simulink model "regulator_PID_obiekt"  (R2014a)
settings: Solver=ode4  StartTime=0.0  StopTime=40  FixedStep=0.01  RelTol=1e-3
undefined symbols (not defined in the file or in its folder): martwa_strefa, T0
undefined symbols (not defined in the file): RTDAC4PCIBaseAddress
settings Model: CovSFcnEnable=on  Creator=Piotr  LastModifiedBy=Praca
settings OptimizationCC: SimCompilerOptimization=off
settings DebuggingCC: UnderspecifiedInitializationDetection=Classic  FrameProcessingCompatibilityMsg=error
settings RTWCC: RTWCompilerOptimization=off

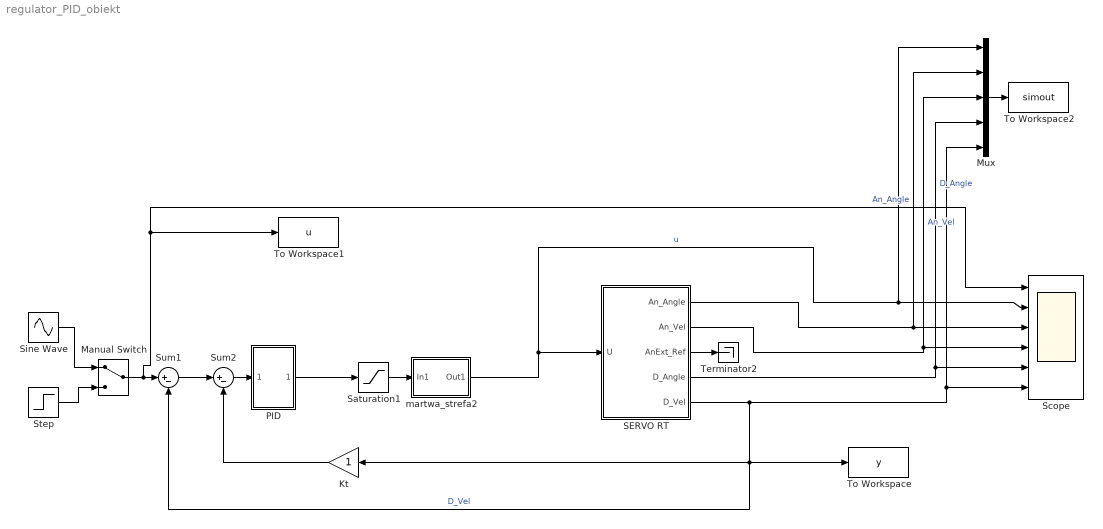
== system regulator_PID_obiekt ==
  Kt : Gain
  Manual Switch : ManualSwitch
  Mux : Mux  Inputs=5
  PID : Subsystem
  SERVO RT : Subsystem
  Saturation1 : Saturate  UpperLimit=1  LowerLimit=-1
  Scope : Scope  NumInputPorts=6
      settings: TimeRange=15  YMin=-0.493553~-4~0~0~0~-5  YMax=-0.446548~4~130~800~70~5  SaveName=obiekt  MaxDataPoints=40000  Decimation=2
  Sine Wave : Sin  SampleTime=0
  Step : Step  After=10  SampleTime=0
  Sum1 : Sum  Inputs=|+-
  Sum2 : Sum  Inputs=|+-
  Terminator2 : Terminator
  To Workspace : ToWorkspace  VariableName=y  SaveFormat=Structure With Time  SampleTime=-1
  To Workspace1 : ToWorkspace  VariableName=u  SaveFormat=Structure With Time  SampleTime=-1
  To Workspace2 : ToWorkspace  VariableName=simout  SaveFormat=Timeseries  SampleTime=-1
  martwa_strefa2 : Subsystem
  wires:
  Sine Wave/1 -> Manual Switch/1
  Step/1 -> Manual Switch/2
  PID/1(Out1) -> Saturation1/1
  Kt/1 -> Sum2/2
  Sum2/1 -> PID/1(In1)
  Sum1/1 -> Sum2/1
  Manual Switch/1 -> To Workspace1/1, Scope/1, Sum1/1
  Saturation1/1 -> martwa_strefa2/1(In1)
  SERVO RT/3(AnExt_Ref) -> Terminator2/1
  SERVO RT/1(An_Angle) -> Scope/3, Mux/2  "An_Angle"
  SERVO RT/2(An_Vel) -> Scope/4, Mux/3  "An_Vel"
  SERVO RT/4(D_Angle) -> Scope/5, Mux/4  "D_Angle"
  SERVO RT/5(D_Vel) -> To Workspace/1, Sum1/2, Kt/1, Scope/6, Mux/5  "D_Vel"
  martwa_strefa2/1(Out1) -> SERVO RT/1(U), Scope/2, Mux/1  "u"
  Mux/1 -> To Workspace2/1

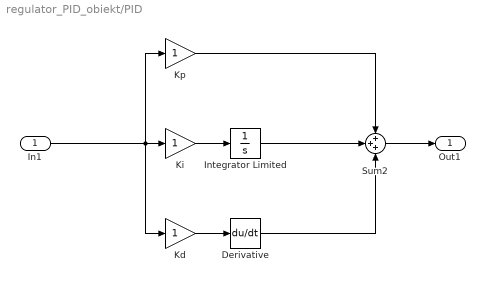
== system regulator_PID_obiekt/PID ==
  In1 : Inport
  Derivative : Derivative
  Integrator Limited : Integrator  LimitOutput=on  UpperSaturationLimit=1  LowerSaturationLimit=-1
  Kd : Gain
  Ki : Gain
  Kp : Gain
  Sum2 : Sum  Inputs=+++
  Out1 : Outport
  wires:
  Kp/1 -> Sum2/1
  Ki/1 -> Integrator Limited/1
  Sum2/1 -> Out1/1
  Kd/1 -> Derivative/1
  In1/1 -> Kp/1, Kd/1, Ki/1
  Derivative/1 -> Sum2/3
  Integrator Limited/1 -> Sum2/2

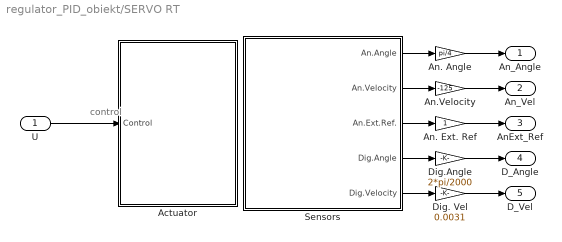
== system regulator_PID_obiekt/SERVO RT ==
  note: control
  U : Inport
  Actuator : Subsystem  mask(Servo Input){BaseAddr=RTDAC4PCIBaseAddress, T0=T0}
      mask prompts: BaseAddr "Base Address"; T0 "Sample Time"
      mask help: RTDAC/PCI Device Driver
      mask Display:
      | plot(0,0,55,85,[15,50,50,50,50,50,50,50,50,50,50,50,50,50,15,25,15],[100,100,90,80,75,70,60,50,40,30,25,20,10,0,0,50,100],[15,25],[50,50],[0,0],[20,80]);
      | text(30,47,'ES 151')
      | text(20,7,'RTDAC/PCI')
  An. Angle : Gain  Gain=pi/4  SaturateOnIntegerOverflow=on  OutDataTypeStr=Inherit: Same as input  ParamDataTypeStr=Inherit: Same as input
  An. Ext. Ref : Gain  SaturateOnIntegerOverflow=on  OutDataTypeStr=Inherit: Same as input  ParamDataTypeStr=Inherit: Same as input
  An.Velocity : Gain  Gain=-125  SaturateOnIntegerOverflow=on  OutDataTypeStr=Inherit: Same as input  ParamDataTypeStr=Inherit: Same as input
  Dig. Vel : Gain  Gain=0.0031  SaturateOnIntegerOverflow=on  OutDataTypeStr=Inherit: Same as input  ParamDataTypeStr=Inherit: Same as input
  Dig.Angle : Gain  Gain=2*pi/2000  SaturateOnIntegerOverflow=on  OutDataTypeStr=Inherit: Same as input  ParamDataTypeStr=Inherit: Same as input
  "Sensors                      " : Subsystem  mask(TRMS Output){BaseAddr=RTDAC4PCIBaseAddress, T0=T0}
      mask prompts: BaseAddr "Base address"; T0 "Sample Time"
      mask help: PCL-812 PG Device Driver
      mask Display:
      | plot(0,0,55,85,85-[55,80,80,80,80,80,80,80,80,80,80,80,80,80,55,50,55],[100,100,90,80,75,70,60,50,40,30,25,20,10,0,0,50,100],[55,55],[100,0],[54,55],[50,50]);
      | text(15,47,'ES 151')
      | text(10,7,'RTDAC/PCI')
  An_Angle : Outport
  An_Vel : Outport  Port=2
  AnExt_Ref : Outport  Port=3
  D_Angle : Outport  Port=4
  D_Vel : Outport  Port=5
  wires:
  An. Angle/1 -> An_Angle/1
  An. Ext. Ref/1 -> AnExt_Ref/1
  Dig. Vel/1 -> D_Vel/1
  An.Velocity/1 -> An_Vel/1
  U/1 -> Actuator/1(Control)
  Dig.Angle/1 -> D_Angle/1
  "Sensors                      "/5(Dig.Velocity) -> Dig. Vel/1
  "Sensors                      "/4(Dig.Angle) -> Dig.Angle/1
  "Sensors                      "/2(An.Velocity) -> An.Velocity/1
  "Sensors                      "/1(An.Angle) -> An. Angle/1
  "Sensors                      "/3(An.Ext.Ref.) -> An. Ext. Ref/1

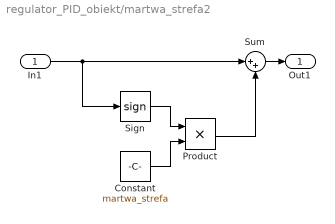
== system regulator_PID_obiekt/martwa_strefa2 ==
  In1 : Inport
  Constant : Constant  Value=martwa_strefa
  Product : Product
  Sign : Signum
  Sum : Sum  Inputs=|++
  Out1 : Outport
  wires:
  In1/1 -> Sum/1, Sign/1
  Product/1 -> Sum/2
  Sign/1 -> Product/1
  Constant/1 -> Product/2
  Sum/1 -> Out1/1

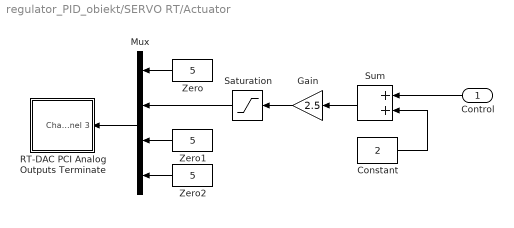
== system regulator_PID_obiekt/SERVO RT/Actuator ==
  Control : Inport
  Constant : Constant  Value=2
  Gain : Gain  Gain=2.5  OutDataTypeStr=Inherit: Same as input  ParamDataTypeStr=Inherit: Same as input
  Mux : Mux
  RT-DAC PCI Analog Outputs Terminate : Subsystem  mask(Analog Output Module){BaseAddress=RTDAC4PCIBaseAddress, VoltRange=-10V - +10V, SetOutputsFlag=on, SetOutputsValue=[0 5 0 0], T0=T0}
      mask prompts: BaseAddress "Base Address:"; VoltRange "Voltage Range"; SetOutputsFlag "Set Outputs At Termination"; SetOutputsValue "Termination Outputs [V]:"; T0 "Sample Time (sec):"
      mask help: RT-DAC PCI Device Driver
      mask Help: Set up each field for your specific hardware configuration.
      mask TypeOptions VoltRange: 0V - +10V | -10V - 0V | -10V - +10V
      mask Display: plot(0,0,100,100,[90,80,80,11,11],[90,90,20,20,80],[11,80],[80,80],[80,80],[20,14],[80,85,85,80],[45,45,66,66],[45,45,74,74],[20,13,13,20],[15,27,27,15,15],[75,75,26,26,75],[33,48,48,33,33],[75,75,55,55,75],[55,55,71,71,55],[55,75,75,55,55],[33,41,41,33,33],[50,50,27,27,50],[48,56,56,48,48],[50,50,27,27,50],[62,70,70,62,62],[50,50,27,27,50])
  Saturation : Saturate  UpperLimit=7.5  LowerLimit=2.5
  Sum : Sum  SaturateOnIntegerOverflow=on  InputSameDT=on  OutDataTypeStr=Inherit: Same as first input
  Zero : Constant  Value=5
  Zero1 : Constant  Value=5
  Zero2 : Constant  Value=5
  wires:
  Constant/1 -> Sum/2
  Sum/1 -> Gain/1
  Gain/1 -> Saturation/1
  Zero1/1 -> Mux/3
  Zero2/1 -> Mux/4
  Mux/1 -> RT-DAC PCI Analog Outputs Terminate/1(Channel 0 Channel 1 Channel 2 Channel 3)
  Saturation/1 -> Mux/2
  Zero/1 -> Mux/1
  Control/1 -> Sum/1

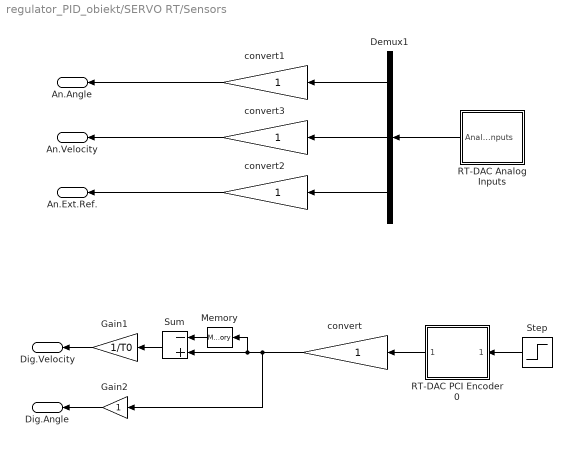
== system regulator_PID_obiekt/SERVO RT/Sensors                       ==
  Demux1 : Demux  Outputs=3
  Gain1 : Gain  Gain=1/T0  SaturateOnIntegerOverflow=on  OutDataTypeStr=Inherit: Same as input  ParamDataTypeStr=Inherit: Same as input
  Gain2 : Gain  SaturateOnIntegerOverflow=on  OutDataTypeStr=Inherit: Same as input  ParamDataTypeStr=Inherit: Same as input
  Memory : Memory
  RT-DAC Analog Inputs : Subsystem  mask(Analog Input Module){BaseAddress=RTDAC4PCIBaseAddress, Chan=[10 11 12], Gain=[1 1 1], T0=T0}
      mask prompts: BaseAddress "Base Address:"; Chan "Channel:"; T0 "Sample Time (sec):"
      mask help: RT-DAC PCI Device Driver
      mask Help: Set up each field for your specific hardware configuration.
      mask Display: plot(0,0,100,100,[90,80,80,11,11],[90,90,20,20,80],[11,80],[80,80],[80,80],[20,14],[80,85,85,80],[45,45,66,66],[45,45,74,74],[20,13,13,20],[15,27,27,15,15],[75,75,26,26,75],[33,48,48,33,33],[75,75,55,55,75],[55,55,71,71,55],[55,75,75,55,55],[33,41,41,33,33],[50,50,27,27,50],[48,56,56,48,48],[50,50,27,27,50],[62,70,70,62,62],[50,50,27,27,50])
  "RT-DAC PCI Encoder 0  " : Subsystem  mask(Incremental Encoders){BaseAddress=RTDAC4PCIBaseAddress, ChannelIdx=0, T0=T0}
      mask prompts: BaseAddress "Base Address:"; ChannelIdx "Channel:"; T0 "Sample Time (sec):"
      mask help: RT-DAC PCI Device Driver
      mask Help: Set up each field for your specific hardware configuration.
      mask TypeOptions ChannelIdx: 0 | 1 | 2 | 3
      mask Display: plot(0,0,100,100,[90,80,80,11,11],[90,90,20,20,80],[11,80],[80,80],[80,80],[20,14],[80,85,85,80],[45,45,66,66],[45,45,74,74],[20,13,13,20],[15,27,27,15,15],[75,75,26,26,75],[33,48,48,33,33],[75,75,55,55,75],[55,55,71,71,55],[55,75,75,55,55],[33,41,41,33,33],[50,50,27,27,50],[48,56,56,48,48],[50,50,27,27,50],[62,70,70,62,62],[50,50,27,27,50])
  Step : Step  Time=T0  Before=1  After=0  SampleTime=0
  Sum : Sum  Inputs=-+  SaturateOnIntegerOverflow=on  InputSameDT=on  OutDataTypeStr=Inherit: Same as first input
  convert : Gain  SaturateOnIntegerOverflow=on  OutDataTypeStr=Inherit: Same as input  ParamDataTypeStr=Inherit: Same as input
  convert1 : Gain  SaturateOnIntegerOverflow=on  OutDataTypeStr=Inherit: Same as input  ParamDataTypeStr=Inherit: Same as input
  convert2 : Gain  SaturateOnIntegerOverflow=on  OutDataTypeStr=Inherit: Same as input  ParamDataTypeStr=Inherit: Same as input
  convert3 : Gain  OutDataTypeStr=Inherit: Same as input  ParamDataTypeStr=Inherit: Same as input
  An.Angle : Outport  InitialOutput=0
  An.Velocity : Outport  Port=2  InitialOutput=0
  An.Ext.Ref. : Outport  Port=3  InitialOutput=0
  Dig.Angle : Outport  Port=4  InitialOutput=0
  Dig.Velocity : Outport  Port=5  InitialOutput=0
  wires:
  Step/1 -> "RT-DAC PCI Encoder 0  "/1(Reset)
  "RT-DAC PCI Encoder 0  "/1(Encoder Counter) -> convert/1
  convert3/1 -> An.Velocity/1
  Demux1/2 -> convert3/1
  convert2/1 -> An.Ext.Ref./1
  Demux1/3 -> convert2/1
  Gain2/1 -> Dig.Angle/1
  Sum/1 -> Gain1/1
  convert/1 -> Gain2/1, Sum/2, Memory/1
  Memory/1 -> Sum/1
  convert1/1 -> An.Angle/1
  Demux1/1 -> convert1/1
  RT-DAC Analog Inputs/1(Analog Inputs) -> Demux1/1
  Gain1/1 -> Dig.Velocity/1

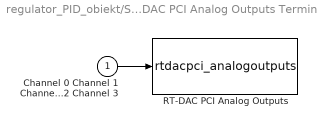
== system regulator_PID_obiekt/SERVO RT/Actuator/RT-DAC PCI Analog Outputs Terminate ==
  Channel 0 Channel 1 Channel 2 Channel 3 : Inport
  "RT-DAC PCI Analog Outputs " : S-Function  FunctionName=rtdacpci_analogoutputs  Parameters=BaseAddress, VoltRange, SetOutputsFlag, SetOutputsValue, T0  EnableBusSupport=off
  wires:
  Channel 0 Channel 1 Channel 2 Channel 3/1 -> "RT-DAC PCI Analog Outputs "/1

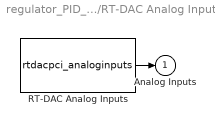
== system regulator_PID_obiekt/SERVO RT/Sensors                      /RT-DAC Analog Inputs ==
  RT-DAC Analog Inputs : S-Function  FunctionName=rtdacpci_analoginputs  Parameters=BaseAddress, Chan, Gain, T0  EnableBusSupport=off
  Analog Inputs : Outport
  wires:
  RT-DAC Analog Inputs/1 -> Analog Inputs/1

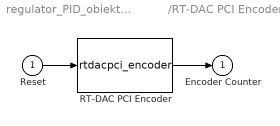
== system regulator_PID_obiekt/SERVO RT/Sensors                      /RT-DAC PCI Encoder 0   ==
  Reset : Inport
  RT-DAC PCI Encoder : S-Function  FunctionName=rtdacpci_encoder  Parameters=BaseAddress, ChannelIdx, T0  EnableBusSupport=off
  Encoder Counter : Outport
  wires:
  Reset/1 -> RT-DAC PCI Encoder/1
  RT-DAC PCI Encoder/1 -> Encoder Counter/1
